simulink model "tank_based_normal_waves_variable"  (R2021b)
settings: Solver=VariableStepAuto  StartTime=0.0  StopTime=20  RelTol=1e-2
values from neighbouring files (symbols this model uses):
  b = 1    [new_parameters.m]
  Be = 5    [new_parameters.m]
  beta = 1e-2    (= 0.01)    [new_parameters.m]
  beta_m = 2*pi*Fc_vel*Ts    (= 0.0628318530718)    [new_parameters.m]
  beta_s = 2*pi*Fc_vel*Ts    (= 0.0628318530718)    [new_parameters.m]
  Bh = 0.02    [new_parameters.m]
  d_m2s = 1    [new_parameters.m]
  d_s2m = 1    [new_parameters.m]
  eQ_m = 2*pi/4096    (= 0.00153398078789)    [new_parameters.m]
  eQ_s = 2*pi/4096    (= 0.00153398078789)    [new_parameters.m]
  Fc_h = 5    [new_parameters.m]
  Filter = 20    [new_parameters.m]
  Hd = 1    [new_parameters.m]
  Hm_init = 1    [new_parameters.m]
  Hs_init = 0    [new_parameters.m]
  Jh = 0.02    [new_parameters.m]
  k_m = 19.34    [new_parameters.m]
  k_s = 19.34    [new_parameters.m]
  Kc2v_m = 4.5    [new_parameters.m]
  Kc2v_s = 4.5    [new_parameters.m]
  Kd_h = 0.5    [new_parameters.m]
  Kd_m = 0.5    [new_parameters.m]
  Kd_s = 0.5    [new_parameters.m]
  Ke = 10    [new_parameters.m]
  Kp_h = 1.2    [new_parameters.m]
  Kp_m = 1    [new_parameters.m]
  Kp_s = 1    [new_parameters.m]
  Kt2c_m = 1.182    [new_parameters.m]
  Kt2c_s = 1.182    [new_parameters.m]
  lArm_m = 0.1    [new_parameters.m]
  lArm_s = 0.1    [new_parameters.m]
  qe = 10    [new_parameters.m]
  tau_m = 1.217    [new_parameters.m]
  tau_s = 1.217    [new_parameters.m]
  tlcAlpha = 0.05    [new_parameters.m]
  Ts = 0.001    [new_parameters.m]
libraries: simulink x2
settings Model: DataTypeOverride=Off  Creator=riccardo  LastModifiedBy=luigi
settings DebuggingCC: IgnoredZcDiagnostic=none  SFMachineParentedDataDiag=warning

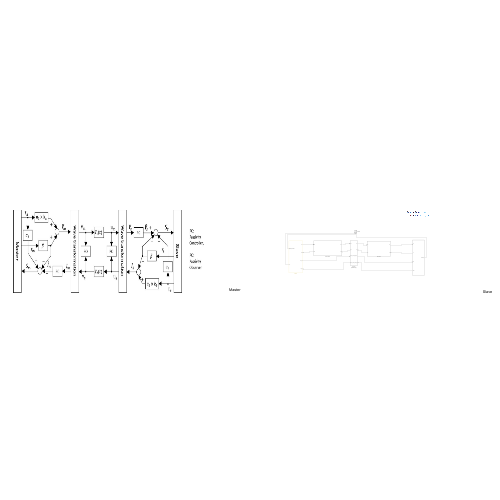
[thumbnail: Simulink's stored preview of the top-level diagram]
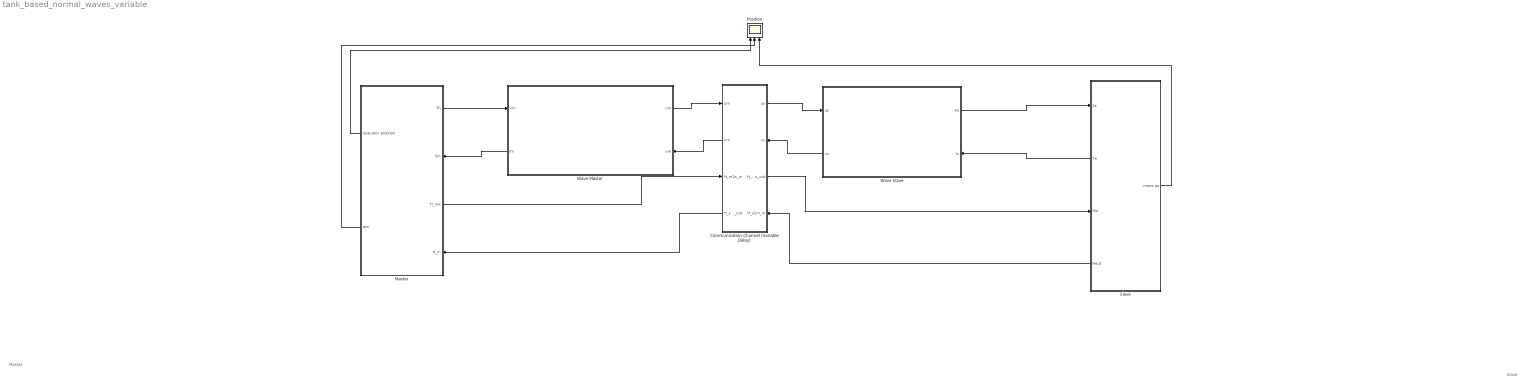
== system tank_based_normal_waves_variable ==
  note: Slave
  note: Master
  Communication Channel (Variable Delay) : Subsystem
      settings: PortSchema="{\"entries\":[{\"content\":{\"sides\":[{\"content\":{\"connectorIds\":[\"In1\",\"Out3\",\"In2\",\"Out4\"]},\"type\":\"ConnectorPlacement.EquallySpacedRectSide\",\"uuid\":\"7e3117e8-bdaa-46b3-a2eb-46f08c8d1fcf\"},{\"content\":{\"connectorIds\":[\"Out1\",\"In3\",\"Out2\",\"In4\"],\"side\":\"RIGHT\"},\"type\":\"ConnectorPlacement.EquallySpacedRectSide\",\"uuid\":\"e52bb446-ae6c-437a-927e-ba88625fbe4c\"},{\"content\":{\"connectorIds\":[],\"side\":\"TOP\"},\"type\":\"ConnectorPlacement.EquallySpacedRectSide\",\"uuid\":\"bd88d442-78a4-4f7f-bea1-c94bcc75de46\"}]},\"type\":\"ConnectorPlacement.EquallySpacedConnector\",\"uuid\":\"e962f433-e609-4b82-bacf-da60dd072235\"}],\"packageUris\":[\"http://schema.mathworks.com/mf0/Connector/R2020b\"],\"version\":\"1.0\"}"
  Master : Subsystem
      settings: PortSchema="{\"entries\":[{\"content\":{\"sides\":[{\"content\":{\"connectorIds\":[\"Out3\",\"Out4\"]},\"type\":\"ConnectorPlacement.EquallySpacedRectSide\",\"uuid\":\"88a440f3-3c17-4ecd-8a7c-55e312326b6c\"},{\"content\":{\"connectorIds\":[\"Out1\",\"In1\",\"Out2\",\"In2\"],\"side\":\"RIGHT\"},\"type\":\"ConnectorPlacement.EquallySpacedRectSide\",\"uuid\":\"1f119ef7-309b-440c-9250-40a12b2cb029\"},{\"content\":{\"connectorIds\":[],\"side\":\"TOP\"},\"type\":\"ConnectorPlacement.EquallySpacedRectSide\",\"uuid\":\"7be3ae0e-cb45-4f37-96af-a21925a9e765\"}]},\"type\":\"ConnectorPlacement.EquallySpacedConnector\",\"uuid\":\"68cc326c-bdcb-4ff9-98f1-957be474a38c\"}],\"packageUris\":[\"http://schema.mathworks.com/mf0/Connector/R2020b\"],\"version\":\"1.0\"}"
  Position : Scope  NumInputPorts=3
  Slave : Subsystem
      settings: PortSchema="{\"entries\":[{\"content\":{\"sides\":[{\"content\":{\"connectorIds\":[\"In1\",\"Out2\",\"In2\",\"Out3\"]},\"type\":\"ConnectorPlacement.EquallySpacedRectSide\",\"uuid\":\"d7867d1a-8ca2-46eb-9cc5-3503a790e4da\"},{\"content\":{\"connectorIds\":[\"Out1\"],\"side\":\"RIGHT\"},\"type\":\"ConnectorPlacement.EquallySpacedRectSide\",\"uuid\":\"2f0413cf-eaaa-4002-929a-cebc19c82c9b\"},{\"content\":{\"connectorIds\":[],\"side\":\"TOP\"},\"type\":\"ConnectorPlacement.EquallySpacedRectSide\",\"uuid\":\"f97ed585-16ab-4e7f-97da-40ff87a224f1\"},{\"content\":{\"connectorIds\":[],\"side\":\"BOTTOM\"},\"type\":\"ConnectorPlacement.EquallySpacedRectSide\",\"uuid\":\"e911c9cd-6707-460b-adc0-d2ecc3cf8bb4\"}]},\"type\":\"ConnectorPlacement.EquallySpacedConnector\",\"uuid\":\"a99d57e5-6d89-49cd-b6f9-976c9398d117\"}],\"packageUris\":[\"http://schema.mathworks.com/mf0/Connector/R2020b\"],\"version\":\"1.0\"}"
  Wave Master : Subsystem
      settings: PortSchema="{\"entries\":[{\"content\":{\"sides\":[{\"content\":{\"connectorIds\":[\"In1\",\"Out2\"]},\"type\":\"ConnectorPlacement.EquallySpacedRectSide\",\"uuid\":\"022537ca-6b1a-446a-b70c-5cc8e9763a20\"},{\"content\":{\"connectorIds\":[\"Out1\",\"In2\"],\"side\":\"RIGHT\"},\"type\":\"ConnectorPlacement.EquallySpacedRectSide\",\"uuid\":\"d2fb6654-cfa2-4536-934e-f2f9b55519fe\"},{\"content\":{\"connectorIds\":[],\"side\":\"TOP\"},\"type\":\"ConnectorPlacement.EquallySpacedRectSide\",\"uuid\":\"40d1266d-c1ee-4ea7-83af-e87fd0883292\"}]},\"type\":\"ConnectorPlacement.EquallySpacedConnector\",\"uuid\":\"3d044237-6122-47a2-8c04-12fd83fac9c7\"}],\"packageUris\":[\"http://schema.mathworks.com/mf0/Connector/R2020b\"],\"version\":\"1.0\"}"
  Wave Slave : Subsystem
      settings: PortSchema="{\"entries\":[{\"content\":{\"sides\":[{\"content\":{\"connectorIds\":[\"In1\",\"Out2\"]},\"type\":\"ConnectorPlacement.EquallySpacedRectSide\",\"uuid\":\"022537ca-6b1a-446a-b70c-5cc8e9763a20\"},{\"content\":{\"connectorIds\":[\"Out1\",\"In2\"],\"side\":\"RIGHT\"},\"type\":\"ConnectorPlacement.EquallySpacedRectSide\",\"uuid\":\"d2fb6654-cfa2-4536-934e-f2f9b55519fe\"},{\"content\":{\"connectorIds\":[],\"side\":\"TOP\"},\"type\":\"ConnectorPlacement.EquallySpacedRectSide\",\"uuid\":\"40d1266d-c1ee-4ea7-83af-e87fd0883292\"}]},\"type\":\"ConnectorPlacement.EquallySpacedConnector\",\"uuid\":\"3d044237-6122-47a2-8c04-12fd83fac9c7\"}],\"packageUris\":[\"http://schema.mathworks.com/mf0/Connector/R2020b\"],\"version\":\"1.0\"}"
  wires:
  Slave/1("meas qs ") -> Position/3
  Master/3("operator position ") -> Position/1
  Master/4(qm) -> Position/2
  Master/1(Th) -> Wave Master/1(Vm)
  Wave Slave/2(vs) -> Communication Channel (Variable Delay)/3(vs)
  Communication Channel (Variable Delay)/1(us) -> Wave Slave/1(us)
  Slave/2(Te) -> Wave Slave/2(Is)
  Wave Master/2(Im) -> Master/1(Sm)
  Wave Master/1(um) -> Communication Channel (Variable Delay)/1(um)
  Communication Channel (Variable Delay)/3(vm) -> Wave Master/2(vm)
  Master/2(H_out) -> Communication Channel (Variable Delay)/2(H_m2s_in)
  Communication Channel (Variable Delay)/4(H_s2m_out) -> Master/2(H_in)
  Wave Slave/1(Vs) -> Slave/1(Ss)
  Slave/3(Hout) -> Communication Channel (Variable Delay)/4(H_s2m_in)
  Communication Channel (Variable Delay)/2(H_m2s_out) -> Slave/2(Hin)

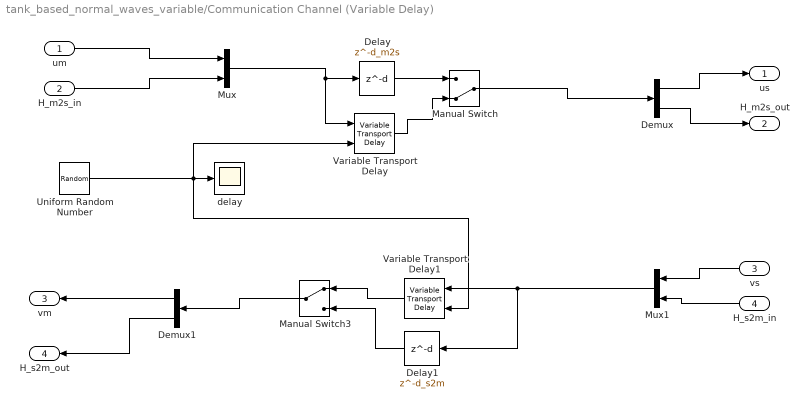
== system tank_based_normal_waves_variable/Communication Channel (Variable Delay) ==
  um : Inport
  H_m2s_in : Inport  Port=2
  vs : Inport  Port=3
  H_s2m_in : Inport  Port=4
  Delay : Delay  DelayLength=d_m2s
  Delay1 : Delay  DelayLength=d_s2m
  Demux : Demux  Outputs=2
  Demux1 : Demux  Outputs=2
  Manual Switch : ManualSwitch  CurrentSetting=0
  Manual Switch3 : ManualSwitch
  Mux : Mux  Inputs=2
  Mux1 : Mux  Inputs=2
  Uniform Random Number : UniformRandomNumber  Minimum=d_m2s-diff  Maximum=d_m2s  SampleTime=1
  Variable Transport Delay : VariableTransportDelay  VariableDelayType=Variable transport delay  MaximumDelay=d_m2s*20  MaximumPoints=100024
  Variable Transport Delay1 : VariableTransportDelay  VariableDelayType=Variable transport delay  MaximumDelay=d_s2m*20  MaximumPoints=100024
  delay : Scope
  us : Outport
  H_m2s_out : Outport  Port=2
  vm : Outport  Port=3
  H_s2m_out : Outport  Port=4
  wires:
  Mux/1 -> Variable Transport Delay/1, Delay/1
  Mux1/1 -> Delay1/1, Variable Transport Delay1/1
  Uniform Random Number/1 -> Variable Transport Delay1/2, delay/1, Variable Transport Delay/2
  Delay/1 -> Manual Switch/1
  Variable Transport Delay/1 -> Manual Switch/2
  Manual Switch/1 -> Demux/1
  Delay1/1 -> Manual Switch3/2
  Manual Switch3/1 -> Demux1/1
  Variable Transport Delay1/1 -> Manual Switch3/1
  um/1 -> Mux/1
  H_m2s_in/1 -> Mux/2
  Demux/1 -> us/1
  Demux/2 -> H_m2s_out/1
  H_s2m_in/1 -> Mux1/2
  vs/1 -> Mux1/1
  Demux1/1 -> vm/1
  Demux1/2 -> H_s2m_out/1

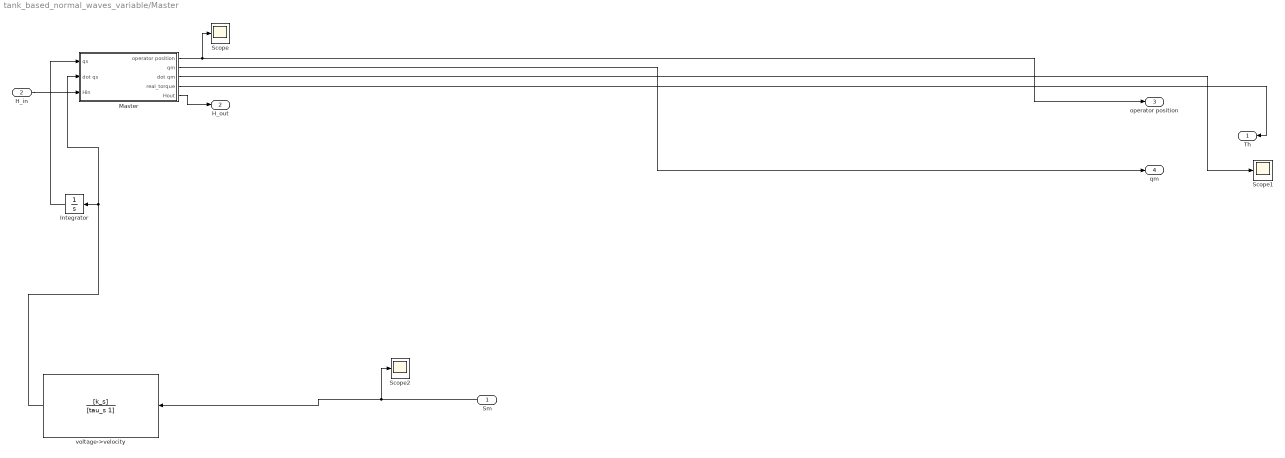
== system tank_based_normal_waves_variable/Master ==
  Sm : Inport
  H_in : Inport  Port=2
  Integrator : Integrator
  Master : Subsystem
  Scope : Scope
  Scope1 : Scope
  Scope2 : Scope
  voltage->velocity : TransferFcn  Numerator=[k_s]  Denominator=[tau_s 1]
  Th : Outport
  H_out : Outport  Port=2
  "operator position " : Outport  Port=3
  qm : Outport  Port=4
  wires:
  Integrator/1 -> Master/1(qs)
  Master/2(qm) -> qm/1
  Master/1("operator position ") -> Scope/1, "operator position "/1
  Master/3(dot qm) -> Scope1/1
  Master/4(real_torque) -> Th/1
  voltage->velocity/1 -> Master/2(dot qs), Integrator/1
  Sm/1 -> Scope2/1, voltage->velocity/1
  Master/5(Hout) -> H_out/1
  H_in/1 -> Master/3(Hin)

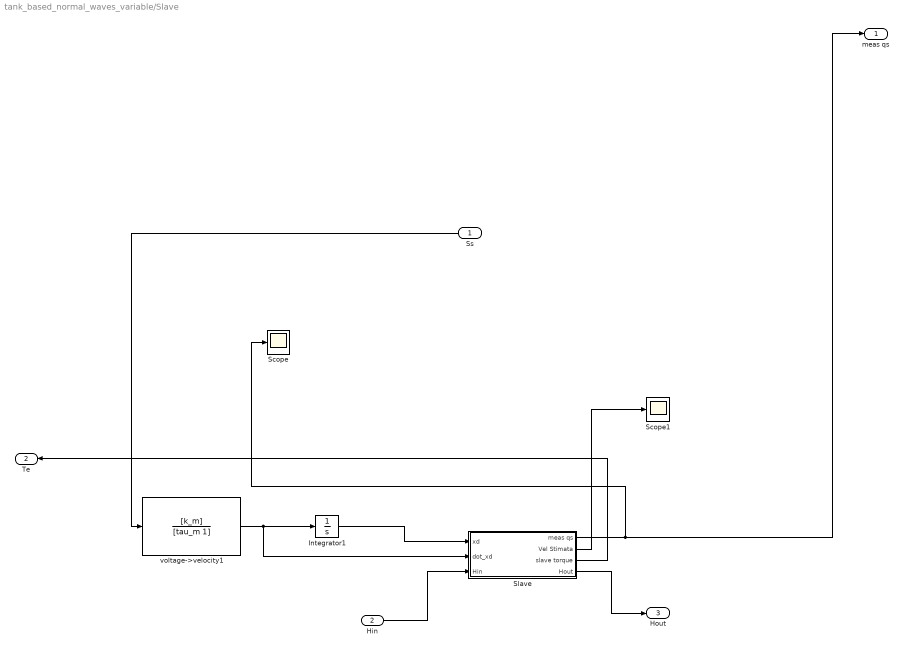
== system tank_based_normal_waves_variable/Slave ==
  Ss : Inport
  Hin : Inport  Port=2
  Integrator1 : Integrator
  Scope : Scope
  Scope1 : Scope
  Slave : Subsystem
  voltage->velocity1 : TransferFcn  Numerator=[k_m]  Denominator=[tau_m 1]
  "meas qs " : Outport
  Te : Outport  Port=2
  Hout : Outport  Port=3
  wires:
  Integrator1/1 -> Slave/1(xd)
  voltage->velocity1/1 -> Integrator1/1, Slave/2(dot_xd)
  Ss/1 -> voltage->velocity1/1
  Slave/1("meas qs ") -> Scope/1, "meas qs "/1
  Slave/3(slave torque) -> Te/1
  Slave/2("Vel Stimata ") -> Scope1/1
  Hin/1 -> Slave/3(Hin)
  Slave/4(Hout) -> Hout/1

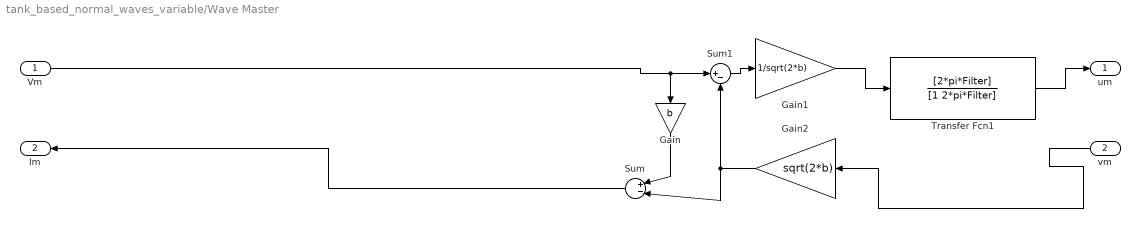
== system tank_based_normal_waves_variable/Wave Master ==
  Vm : Inport
  vm : Inport  Port=2
  Gain : Gain  Gain=b
  Gain1 : Gain  Gain=1/sqrt(2*b)
  Gain2 : Gain  Gain=sqrt(2*b)
  Sum : Sum  Inputs=|+-|
  Sum1 : Sum  Inputs=|+-
  Transfer Fcn1 : TransferFcn  Numerator=[2*pi*Filter]  Denominator=[1 2*pi*Filter]
  um : Outport
  Im : Outport  Port=2
  wires:
  Transfer Fcn1/1 -> um/1
  Gain1/1 -> Transfer Fcn1/1
  Vm/1 -> Sum1/1, Gain/1
  Gain/1 -> Sum/1
  Gain2/1 -> Sum1/2, Sum/2
  Sum/1 -> Im/1
  Sum1/1 -> Gain1/1
  vm/1 -> Gain2/1

== system tank_based_normal_waves_variable/Wave Slave ==
  us : Inport
  Is : Inport  Port=2
  Gain : Gain  Gain=1/b
  Gain3 : Gain  Gain=2/sqrt(2*b)
  Gain5 : Gain  Gain=2/sqrt(2*b)
  Sum : Sum  Inputs=|+-
  Sum1 : Sum  Inputs=|+-
  Vs : Outport
  vs : Outport  Port=2
  wires:
  us/1 -> Sum1/1, Gain3/1
  Is/1 -> Gain5/1, Gain/1
  Sum/1 -> Vs/1
  Gain/1 -> Sum/2
  Gain3/1 -> Sum/1
  Gain5/1 -> Sum1/2
  Sum1/1 -> vs/1

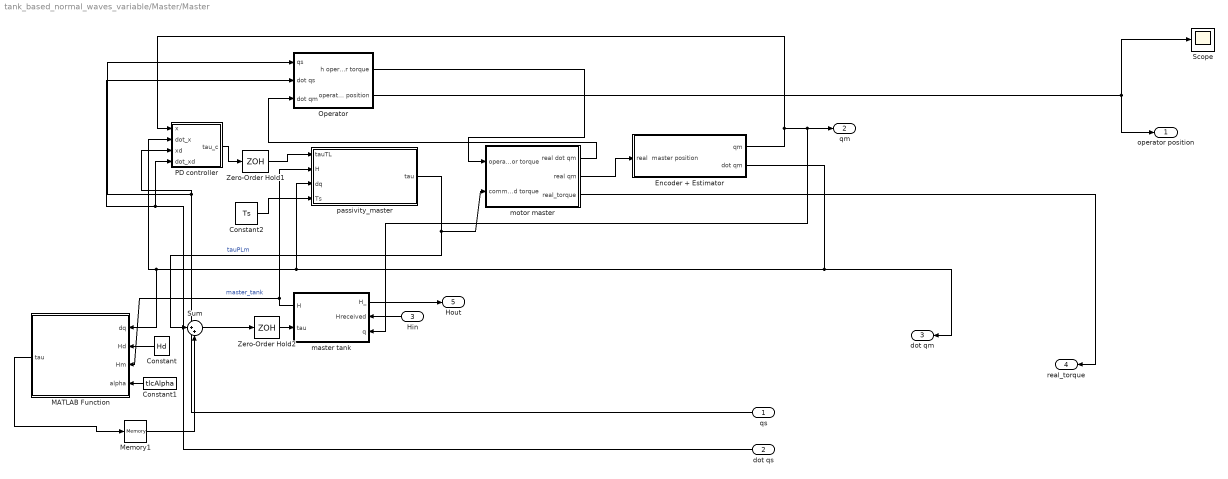
== system tank_based_normal_waves_variable/Master/Master ==
  qs : Inport
  dot qs : Inport  Port=2
  Hin : Inport  Port=3
  Constant : Constant  Value=Hd
  Constant1 : Constant  Value=tlcAlpha
  Constant2 : Constant  Value=Ts
  Encoder + Estimator : Subsystem
  MATLAB Function : MATLAB Function  TreatAsAtomicUnit=on
  Memory1 : Memory
  Operator : Subsystem
  PD controller : Subsystem
  Scope : Scope
  Sum : Sum  Inputs=|++
  Zero-Order Hold1 : ZeroOrderHold  SampleTime=Ts
  Zero-Order Hold2 : ZeroOrderHold  SampleTime=Ts
  master tank : Subsystem
      settings: PortSchema="{\"entries\":[{\"content\":{\"sides\":[{\"content\":{\"connectorIds\":[\"Out2\",\"In1\",\"In2\"]},\"type\":\"ConnectorPlacement.EquallySpacedRectSide\",\"uuid\":\"482b0a11-f044-49fa-a74d-4dac8b5b787b\"},{\"content\":{\"connectorIds\":[\"Out1\",\"In3\"],\"side\":\"RIGHT\"},\"type\":\"ConnectorPlacement.EquallySpacedRectSide\",\"uuid\":\"b0c369ed-ae40-43d8-b393-bca9f7720d62\"},{\"content\":{\"connectorIds\":[],\"side\":\"TOP\"},\"type\":\"ConnectorPlacement.EquallySpacedRectSide\",\"uuid\":\"ff021616-d6aa-4c0a-874b-a9ebe947c92c\"},{\"content\":{\"connectorIds\":[],\"side\":\"BOTTOM\"},\"type\":\"ConnectorPlacement.EquallySpacedRectSide\",\"uuid\":\"4e18ee96-bca7-41b6-9abb-5b593b41c296\"},{\"content\":{\"connectorIds\":[],\"side\":\"HIDDEN\"},\"type\":\"ConnectorPlacement.EquallySpacedRectSide\",\"uuid\":\"be815b34-35c7-4c6f-8c8b-4a812b3d12e9\"}]},\"type\":\"ConnectorPlacement.EquallySpacedConnector\",\"uuid\":\"78552b8a-5f1c-4815-a807-de98f58b7f2e\"}],\"packageUris\":[\"http://schema.mathworks.com/mf0/Connector/R2020b\"],\"version\":\"1.0\"}"
  motor master : Subsystem
  passivity_master : MATLAB Function  TreatAsAtomicUnit=on
  "operator position " : Outport
  qm : Outport  Port=2
  dot qm : Outport  Port=3
  real_torque : Outport  Port=4
  Hout : Outport  Port=5
  wires:
  motor master/1(real dot qm) -> Operator/3(dot qm)
  PD controller/1(tau_c) -> Zero-Order Hold1/1
  qs/1 -> PD controller/3(xd), Operator/1(qs)
  motor master/2(real qm) -> Encoder + Estimator/1(real  master position)
  Operator/1(h operator torque) -> motor master/1(operator torque)
  Encoder + Estimator/2(dot qm) -> MATLAB Function/1(dq), PD controller/2(dot_x), passivity_master/3(dq), dot qm/1
  motor master/3(real_torque) -> real_torque/1
  Operator/2("operator position ") -> Scope/1, "operator position "/1
  Encoder + Estimator/1(qm) -> master tank/2(q), qm/1, PD controller/1(x)
  Zero-Order Hold1/1 -> passivity_master/1(tauTL)
  Hin/1 -> master tank/1(Hreceived)
  MATLAB Function/1(tau) -> Memory1/1
  passivity_master/1(tau) -> Sum/1, motor master/2(command torque)  "tauPLm"
  Zero-Order Hold2/1 -> master tank/3(tau)
  master tank/1(H) -> passivity_master/2(H), MATLAB Function/3(Hm)  "master_tank"
  Constant/1 -> MATLAB Function/2(Hd)
  Constant1/1 -> MATLAB Function/4(alpha)
  dot qs/1 -> PD controller/4(dot_xd), Operator/2(dot qs)
  master tank/2(H_) -> Hout/1
  Constant2/1 -> passivity_master/4(Ts)
  Memory1/1 -> Sum/2
  Sum/1 -> Zero-Order Hold2/1

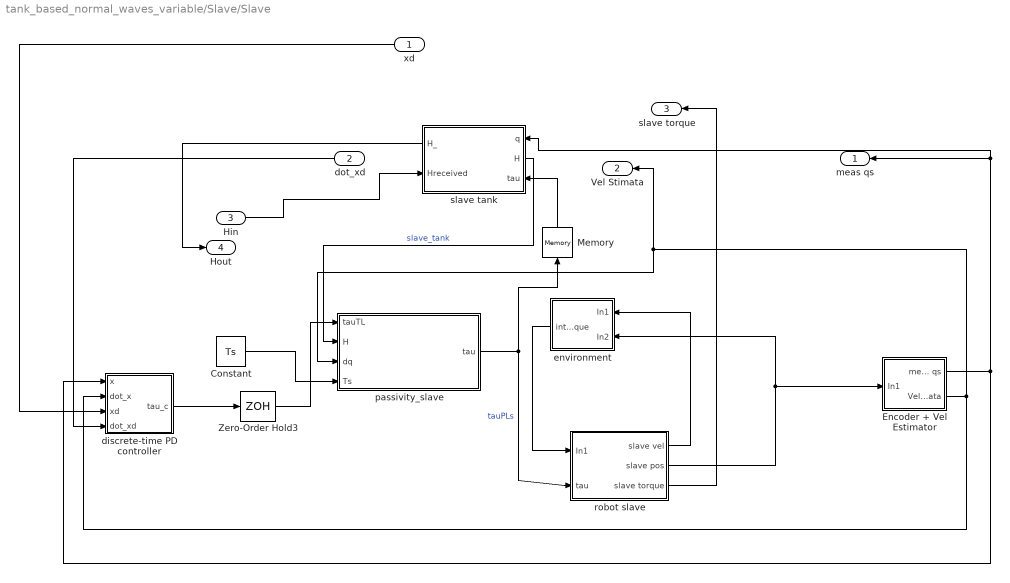
== system tank_based_normal_waves_variable/Slave/Slave ==
  xd : Inport
  dot_xd : Inport  Port=2
  Hin : Inport  Port=3
  Constant : Constant  Value=Ts
  "Encoder + Vel Estimator " : Subsystem
  Memory : Memory
  Zero-Order Hold3 : ZeroOrderHold  SampleTime=Ts
  discrete-time PD controller : Subsystem
  "environment " : Subsystem
  passivity_slave : MATLAB Function  TreatAsAtomicUnit=on
  "robot slave " : Subsystem
  slave tank : Subsystem
      settings: PortSchema="{\"entries\":[{\"content\":{\"sides\":[{\"content\":{\"connectorIds\":[\"In1\",\"Out2\",\"In2\"]},\"type\":\"ConnectorPlacement.EquallySpacedRectSide\",\"uuid\":\"482b0a11-f044-49fa-a74d-4dac8b5b787b\"},{\"content\":{\"connectorIds\":[\"Out1\",\"In3\"],\"side\":\"RIGHT\"},\"type\":\"ConnectorPlacement.EquallySpacedRectSide\",\"uuid\":\"b0c369ed-ae40-43d8-b393-bca9f7720d62\"},{\"content\":{\"connectorIds\":[],\"side\":\"TOP\"},\"type\":\"ConnectorPlacement.EquallySpacedRectSide\",\"uuid\":\"ff021616-d6aa-4c0a-874b-a9ebe947c92c\"},{\"content\":{\"connectorIds\":[],\"side\":\"BOTTOM\"},\"type\":\"ConnectorPlacement.EquallySpacedRectSide\",\"uuid\":\"4e18ee96-bca7-41b6-9abb-5b593b41c296\"},{\"content\":{\"connectorIds\":[],\"side\":\"HIDDEN\"},\"type\":\"ConnectorPlacement.EquallySpacedRectSide\",\"uuid\":\"be815b34-35c7-4c6f-8c8b-4a812b3d12e9\"}]},\"type\":\"ConnectorPlacement.EquallySpacedConnector\",\"uuid\":\"78552b8a-5f1c-4815-a807-de98f58b7f2e\"}],\"packageUris\":[\"http://schema.mathworks.com/mf0/Connector/R2020b\"],\"version\":\"1.0\"}"
  "meas qs " : Outport
  "Vel Stimata " : Outport  Port=2
  slave torque : Outport  Port=3
  Hout : Outport  Port=4
  wires:
  "robot slave "/1(slave vel) -> "environment "/1(In1)
  "robot slave "/2(slave pos) -> "environment "/2(In2), "Encoder + Vel Estimator "/1(In1)
  "Encoder + Vel Estimator "/1("meas qs ") -> slave tank/1(q), "meas qs "/1, discrete-time PD controller/1(x)
  Zero-Order Hold3/1 -> passivity_slave/1(tauTL)
  "Encoder + Vel Estimator "/2("Vel Stimata ") -> "Vel Stimata "/1, passivity_slave/3(dq), discrete-time PD controller/2(dot_x)
  discrete-time PD controller/1(tau_c) -> Zero-Order Hold3/1
  "environment "/1("interaction torque ") -> "robot slave "/1(In1)
  dot_xd/1 -> discrete-time PD controller/4(dot_xd)
  xd/1 -> discrete-time PD controller/3(xd)
  "robot slave "/3(slave torque) -> slave torque/1
  Hin/1 -> slave tank/3(Hreceived)
  Constant/1 -> passivity_slave/4(Ts)
  passivity_slave/1(tau) -> "robot slave "/2(tau), Memory/1  "tauPLs"
  slave tank/1(H_) -> Hout/1
  slave tank/2(H) -> passivity_slave/2(H)  "slave_tank"
  Memory/1 -> slave tank/2(tau)

== system tank_based_normal_waves_variable/Master/Master/Encoder + Estimator ==
  real  master position : Inport
  Constant : Constant  Value=eQ_m
  Sum : Sum  Inputs=++|
  Velocity estimator : Subsystem
  Zero-Order Hold : ZeroOrderHold  SampleTime=Ts
  noise : MATLAB Function  TreatAsAtomicUnit=on
  qm : Outport
  dot qm : Outport  Port=2
  wires:
  real  master position/1 -> Zero-Order Hold/1
  Zero-Order Hold/1 -> Sum/2
  Sum/1 -> qm/1, Velocity estimator/1(pos misurata)
  Constant/1 -> noise/1(delta_q)
  Velocity estimator/1(Vel stimata) -> dot qm/1
  noise/1(error) -> Sum/1

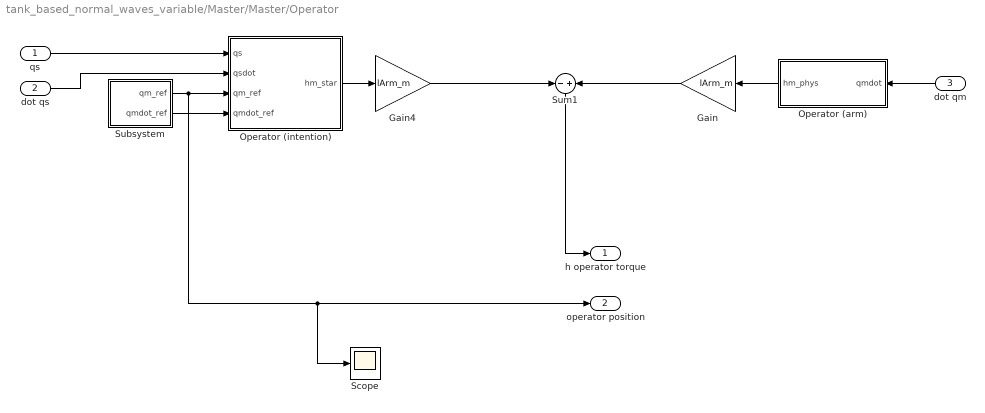
== system tank_based_normal_waves_variable/Master/Master/Operator ==
  qs : Inport
  dot qs : Inport  Port=2
  dot qm : Inport  Port=3
  Gain : Gain  Gain=lArm_m
  Gain4 : Gain  Gain=lArm_m
  Operator (arm) : Subsystem
  Operator (intention) : Subsystem
  Scope : Scope
  Subsystem : Subsystem
  Sum1 : Sum  Inputs=-+
  h operator torque : Outport
  "operator position " : Outport  Port=2
  wires:
  Sum1/1 -> h operator torque/1
  Operator (arm)/1(hm_phys) -> Gain/1
  dot qm/1 -> Operator (arm)/1(qmdot)
  Subsystem/2(qmdot_ref) -> Operator (intention)/4(qmdot_ref)
  Operator (intention)/1(hm_star) -> Gain4/1
  dot qs/1 -> Operator (intention)/2(qsdot)
  Gain4/1 -> Sum1/1
  Gain/1 -> Sum1/2
  Subsystem/1(qm_ref) -> Scope/1, "operator position "/1, Operator (intention)/3(qm_ref)
  qs/1 -> Operator (intention)/1(qs)

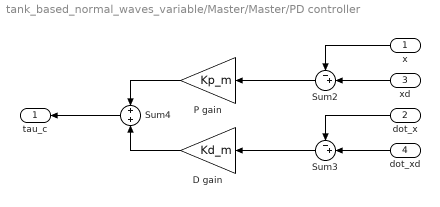
== system tank_based_normal_waves_variable/Master/Master/PD controller ==
  x : Inport
  dot_x : Inport  Port=2
  xd : Inport  Port=3
  dot_xd : Inport  Port=4
  D gain : Gain  Gain=Kd_m
  P gain : Gain  Gain=Kp_m
  Sum2 : Sum  Inputs=-+|
  Sum3 : Sum  Inputs=-+|
  Sum4 : Sum
  tau_c : Outport  VectorParamsAs1DForOutWhenUnconnected=off
  wires:
  D gain/1 -> Sum4/2
  dot_x/1 -> Sum3/1
  dot_xd/1 -> Sum3/2
  x/1 -> Sum2/1
  xd/1 -> Sum2/2
  Sum3/1 -> D gain/1
  P gain/1 -> Sum4/1
  Sum4/1 -> tau_c/1
  Sum2/1 -> P gain/1

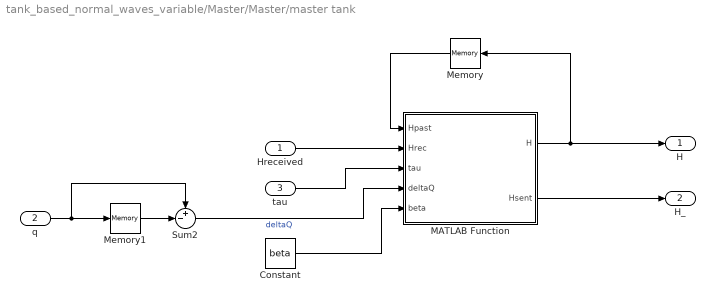
== system tank_based_normal_waves_variable/Master/Master/master tank ==
  Hreceived : Inport
  q : Inport  Port=2
  tau : Inport  Port=3
  Constant : Constant  Value=beta
  MATLAB Function : MATLAB Function  TreatAsAtomicUnit=on
  Memory : Memory  InitialCondition=Hm_init
  Memory1 : Memory
  Sum2 : Sum  Inputs=+-|
  H : Outport
  H_ : Outport  Port=2
  wires:
  Memory1/1 -> Sum2/2
  q/1 -> Memory1/1, Sum2/1
  MATLAB Function/2(Hsent) -> H_/1
  Constant/1 -> MATLAB Function/5(beta)
  Sum2/1 -> MATLAB Function/4(deltaQ)  "deltaQ"
  Hreceived/1 -> MATLAB Function/2(Hrec)
  tau/1 -> MATLAB Function/3(tau)
  MATLAB Function/1(H) -> Memory/1, H/1
  Memory/1 -> MATLAB Function/1(Hpast)

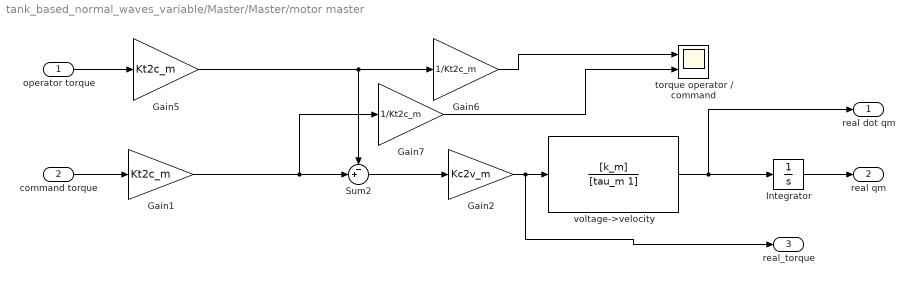
== system tank_based_normal_waves_variable/Master/Master/motor master ==
  operator torque : Inport
  command torque : Inport  Port=2
  Gain1 : Gain  Gain=Kt2c_m
  Gain2 : Gain  Gain=Kc2v_m
  Gain5 : Gain  Gain=Kt2c_m
  Gain6 : Gain  Gain=1/Kt2c_m
  Gain7 : Gain  Gain=1/Kt2c_m
  Integrator : Integrator
  Sum2 : Sum  Inputs=-+|
  torque operator / command : Scope  NumInputPorts=2
  voltage->velocity : TransferFcn  Numerator=[k_m]  Denominator=[tau_m 1]
  real dot qm : Outport
  real qm : Outport  Port=2
  real_torque : Outport  Port=3
  wires:
  Gain7/1 -> torque operator / command/2
  operator torque/1 -> Gain5/1
  Gain2/1 -> real_torque/1, voltage->velocity/1
  Gain1/1 -> Gain7/1, Sum2/2
  Integrator/1 -> real qm/1
  command torque/1 -> Gain1/1
  Gain6/1 -> torque operator / command/1
  voltage->velocity/1 -> real dot qm/1, Integrator/1
  Sum2/1 -> Gain2/1
  Gain5/1 -> Sum2/1, Gain6/1

== system tank_based_normal_waves_variable/Slave/Slave/Encoder + Vel Estimator  ==
  In1 : Inport
  Constant : Constant  Value=eQ_s
  Subsystem : Subsystem
  Sum : Sum  Inputs=++|
  Zero-Order Hold : ZeroOrderHold  SampleTime=Ts
  noise : MATLAB Function  TreatAsAtomicUnit=on
  "meas qs " : Outport
  "Vel Stimata " : Outport  Port=2
  wires:
  Constant/1 -> noise/1(delta_q)
  In1/1 -> Zero-Order Hold/1
  noise/1(error) -> Sum/1
  Zero-Order Hold/1 -> Sum/2
  Sum/1 -> "meas qs "/1, Subsystem/1(pos misurata)
  Subsystem/1(Vel stimata) -> "Vel Stimata "/1

== system tank_based_normal_waves_variable/Slave/Slave/discrete-time PD controller ==
  x : Inport
  dot_x : Inport  Port=2
  xd : Inport  Port=3
  dot_xd : Inport  Port=4
  D gain : Gain  Gain=Kd_s
  P gain : Gain  Gain=Kp_s
  Sum2 : Sum  Inputs=-+|
  Sum3 : Sum  Inputs=-+|
  Sum4 : Sum
  tau_c : Outport  VectorParamsAs1DForOutWhenUnconnected=off
  wires:
  D gain/1 -> Sum4/2
  dot_x/1 -> Sum3/1
  dot_xd/1 -> Sum3/2
  x/1 -> Sum2/1
  xd/1 -> Sum2/2
  Sum3/1 -> D gain/1
  P gain/1 -> Sum4/1
  Sum4/1 -> tau_c/1
  Sum2/1 -> P gain/1

== system tank_based_normal_waves_variable/Slave/Slave/environment  ==
  note: qs
  note: qdot
  In1 : Inport
  In2 : Inport  Port=2
  Environment : Subsystem
  Gain : Gain  Gain=lArm_s
  "interaction torque " : Outport
  wires:
  In2/1 -> Environment/2(qs)
  Environment/1(fe) -> Gain/1
  In1/1 -> Environment/1(qsdot)
  Gain/1 -> "interaction torque "/1

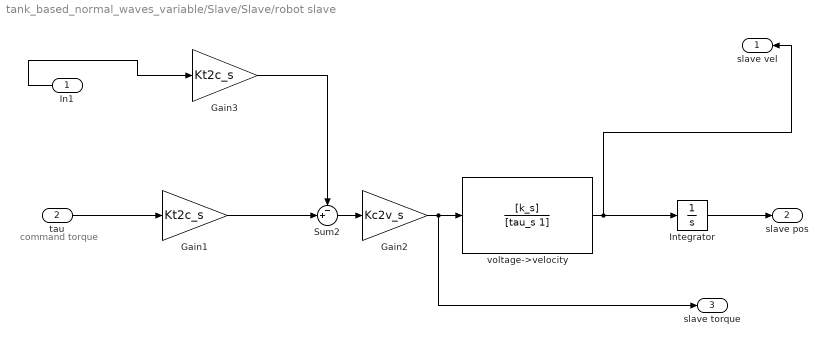
== system tank_based_normal_waves_variable/Slave/Slave/robot slave  ==
  note: command torque
  In1 : Inport
  tau : Inport  Port=2
  Gain1 : Gain  Gain=Kt2c_s
  Gain2 : Gain  Gain=Kc2v_s
  Gain3 : Gain  Gain=Kt2c_s
  Integrator : Integrator
  Sum2 : Sum  Inputs=-+|
  voltage->velocity : TransferFcn  Numerator=[k_s]  Denominator=[tau_s 1]
  slave vel : Outport
  slave pos : Outport  Port=2
  slave torque : Outport  Port=3
  wires:
  Gain2/1 -> slave torque/1, voltage->velocity/1
  Gain3/1 -> Sum2/1
  voltage->velocity/1 -> slave vel/1, Integrator/1
  Gain1/1 -> Sum2/2
  Sum2/1 -> Gain2/1
  Integrator/1 -> slave pos/1
  In1/1 -> Gain3/1
  tau/1 -> Gain1/1

== system tank_based_normal_waves_variable/Slave/Slave/slave tank ==
  q : Inport
  tau : Inport  Port=2
  Hreceived : Inport  Port=3
  Constant : Constant  Value=beta
  MATLAB Function : MATLAB Function  TreatAsAtomicUnit=on
  Memory : Memory  InitialCondition=Hs_init
  Memory1 : Memory
  Sum2 : Sum  Inputs=+-|
  H_ : Outport
  H : Outport  Port=2
  wires:
  Memory1/1 -> Sum2/2
  MATLAB Function/2(Hsent) -> H_/1
  Constant/1 -> MATLAB Function/5(beta)
  Sum2/1 -> MATLAB Function/4(deltaQ)  "deltaQ"
  Hreceived/1 -> MATLAB Function/2(Hrec)
  tau/1 -> MATLAB Function/3(tau)
  MATLAB Function/1(H) -> Memory/1, H/1
  Memory/1 -> MATLAB Function/1(Hpast)
  q/1 -> Memory1/1, Sum2/1

== system tank_based_normal_waves_variable/Master/Master/Encoder + Estimator/Velocity estimator ==
  pos misurata : Inport
  Difference : simulink/Discrete/Difference  ICPrevInput=0.0  OutMin=[]  OutMax=[]  OutDataType=fixdt(1, 16)  OutScaling=2^-10  DoSatur=off
  Filtro passabasso : DiscreteTransferFcn  Numerator=[beta_m 0]  Denominator=[1 -(1-beta_m)]  SampleTime=Ts
  Gain2 : Gain  Gain=1/Ts
  Vel stimata : Outport  VectorParamsAs1DForOutWhenUnconnected=off
  wires:
  Gain2/1 -> Filtro passabasso/1
  pos misurata/1 -> Difference/1
  Difference/1 -> Gain2/1
  Filtro passabasso/1 -> Vel stimata/1  "Velocità  stimata"

== system tank_based_normal_waves_variable/Master/Master/Operator/Operator (arm) ==
  note: force
  qmdot : Inport
  Derivative : Derivative  CoefficientInTFapproximation=0.001
  Gain1 : Gain  Gain=Jh
  Gain2 : Gain  Gain=Bh
  Sum : Sum  Inputs=+|+
  hm_phys : Outport  VectorParamsAs1DForOutWhenUnconnected=off
  wires:
  qmdot/1 -> Gain2/1, Derivative/1
  Sum/1 -> hm_phys/1
  Derivative/1 -> Gain1/1
  Gain2/1 -> Sum/1
  Gain1/1 -> Sum/2

== system tank_based_normal_waves_variable/Master/Master/Operator/Operator (intention) ==
  qs : Inport
  qsdot : Inport  Port=2
  qm_ref : Inport  Port=3
  qmdot_ref : Inport  Port=4
  Gain3 : Gain  Gain=Kp_h
  Gain4 : Gain  Gain=Kd_h
  Sum1 : Sum  Inputs=+|-
  Sum2 : Sum  Inputs=+|-
  Sum3 : Sum  Inputs=+|+
  hm_star : Outport  VectorParamsAs1DForOutWhenUnconnected=off
  wires:
  qs/1 -> Sum1/2
  qm_ref/1 -> Sum1/1
  qmdot_ref/1 -> Sum2/1
  Sum1/1 -> Gain3/1
  qsdot/1 -> Sum2/2
  Sum2/1 -> Gain4/1
  Gain4/1 -> Sum3/1
  Gain3/1 -> Sum3/2
  Sum3/1 -> hm_star/1

== system tank_based_normal_waves_variable/Master/Master/Operator/Subsystem ==
  Derivative1 : Derivative  CoefficientInTFapproximation=0.001
  Manual Switch : ManualSwitch
  Sine Wave : Sin  SampleTime=0
  Step : Step  SampleTime=0
  low-pass filter : TransferFcn  Numerator=[2*pi*Fc_h]  Denominator=[1 2*pi*Fc_h]
  qm_ref : Outport
  qmdot_ref : Outport  Port=2
  wires:
  low-pass filter/1 -> Manual Switch/2
  Manual Switch/1 -> qm_ref/1, Derivative1/1
  Derivative1/1 -> qmdot_ref/1  "qmdot_ref"
  Step/1 -> low-pass filter/1
  Sine Wave/1 -> Manual Switch/1

== system tank_based_normal_waves_variable/Slave/Slave/Encoder + Vel Estimator /Subsystem ==
  pos misurata : Inport
  Difference : simulink/Discrete/Difference  ICPrevInput=0.0  OutMin=[]  OutMax=[]  OutDataType=fixdt(1, 16)  OutScaling=2^-10  DoSatur=off
  Filtro passabasso : DiscreteTransferFcn  Numerator=[beta_s 0]  Denominator=[1 -(1-beta_s)]  SampleTime=Ts
  Gain2 : Gain  Gain=1/Ts
  Vel stimata : Outport  VectorParamsAs1DForOutWhenUnconnected=off
  wires:
  Gain2/1 -> Filtro passabasso/1
  pos misurata/1 -> Difference/1
  Difference/1 -> Gain2/1
  Filtro passabasso/1 -> Vel stimata/1  "Velocità  stimata"

== system tank_based_normal_waves_variable/Slave/Slave/environment /Environment ==
  note: force
  qsdot : Inport
  qs : Inport  Port=2
  Constant : Constant  Value=qe  SampleTime=0
  c1 : Constant  Value=Be  SampleTime=0
  c2 : Constant  Value=Ke  SampleTime=0
  env : MATLAB Function  TreatAsAtomicUnit=on
  fe : Outport  VectorParamsAs1DForOutWhenUnconnected=off
  wires:
  Constant/1 -> env/3(qe)
  c1/1 -> env/2(Be)
  c2/1 -> env/1(Ke)
  qs/1 -> env/4(qs)
  qsdot/1 -> env/5(qsdot)
  env/1(fE) -> fe/1

== matlab function tank_based_normal_waves_variable/Slave/Slave/Encoder + Vel Estimator /noise ==
  data: delta_q input; error output
function error = noise_measurement(delta_q)
if randn(1)>0
   error = delta_q;
else
    error = -delta_q;
end

== matlab function tank_based_normal_waves_variable/Master/Master/Encoder + Estimator/noise ==
  data: delta_q input; error output
function error = noise_measurement(delta_q)
if randn(1)>0
   error = delta_q;
else
    error = -delta_q;
end

== matlab function tank_based_normal_waves_variable/Master/Master/master tank/MATLAB Function ==
  data: Hpast input; H output; Hrec input; tau input; deltaQ input; beta input; Hsent output
function [H,Hsent] = tank(Hpast, Hrec, tau, deltaQ, beta)
Hused = tau*deltaQ;
H = Hpast+Hrec-Hused;    
Hsent = H*beta;
H = H-Hsent;

== matlab function tank_based_normal_waves_variable/Master/Master/MATLAB Function ==
  data: dq input; tau output; Hd input; Hm input; alpha input
function tau = tauTLC(dq, Hd, Hm, alpha)
%tank level controller
%Energy Tanks slide 16
if Hd <= Hm
    d = 0;
else
    d = alpha*(Hd-Hm);
end
tau = -d*dq;

== matlab function tank_based_normal_waves_variable/Master/Master/passivity_master ==
  data: tauTL input; H input; tau output; dq input; Ts input
function tau = tauPL(tauTL, H, dq,Ts)
%saturation and control torque 
%slide 19 tau max 1 2
if H<= 0
    tauMax1 = 0;
else
    tauMax1 = tauTL;
end
tauMax2 = H/(dq*Ts);

%limited torque computed by the passivity layer based on τauTL
tau = sign(tauTL)*min([abs(tauMax1),abs(tauMax2)]);

== matlab function tank_based_normal_waves_variable/Slave/Slave/passivity_slave ==
  data: tauTL input; H input; tau output; dq input; Ts input
function tau = tauPL(tauTL, H, dq,Ts)
if H<= 0
    tauMax1 = 0;
else
    tauMax1 = tauTL;
end
tauMax2 = H/(dq*Ts);
tau = sign(tauTL)*min([abs(tauMax1),abs(tauMax2)]);

== matlab function tank_based_normal_waves_variable/Slave/Slave/slave tank/MATLAB Function ==
  data: Hpast input; H output; Hrec input; tau input; deltaQ input; beta input; Hsent output
function [H,Hsent] = tank(Hpast, Hrec, tau, deltaQ, beta)
Hused = tau*deltaQ;
H = Hpast+Hrec-Hused;    
Hsent = H*beta;
H = H-Hsent;

== matlab function tank_based_normal_waves_variable/Slave/Slave/environment /Environment/env ==
  data: Ke input; Be input; qe input; qs input; fE output; qsdot input
function fE  = environment(Ke, Be, qe, qs, qsdot)
if qs > qe
   fE = Ke * (qs - qe) + Be * qsdot;
else
   fE = 0;
end
